simulink model "chap2_8sim"  (R2016a)
settings: Solver=VariableStepAuto  StartTime=0.0  StopTime=10.0  RelTol=1e-3
settings Model: Creator=zhanghankui  LastModifiedBy=zhanghankui

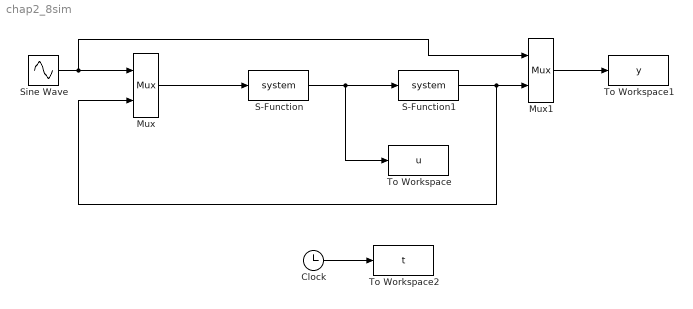
== system chap2_8sim ==
  Clock : Clock
  Mux : Mux  Inputs=2
  Mux1 : Mux  Inputs=2
  S-Function : S-Function  SFunctionDeploymentMode=off  EnableBusSupport=off
  S-Function1 : S-Function  SFunctionDeploymentMode=off  EnableBusSupport=off
  Sine Wave : Sin  SampleTime=0
  To Workspace : ToWorkspace  VariableName=u  SaveFormat=Timeseries  SampleTime=-1
  To Workspace1 : ToWorkspace  VariableName=y  SaveFormat=Timeseries  SampleTime=-1
  To Workspace2 : ToWorkspace  VariableName=t  SaveFormat=Timeseries  SampleTime=-1
  wires:
  Sine Wave/1 -> Mux1/1, Mux/1
  Mux/1 -> S-Function/1
  S-Function/1 -> To Workspace/1, S-Function1/1
  S-Function1/1 -> Mux/2, Mux1/2
  Mux1/1 -> To Workspace1/1
  Clock/1 -> To Workspace2/1
